simulink model "Iris_DeePC_Control_Gazebo_hyper"  (R2022a)
settings: Solver=VariableStepAuto  StartTime=0.0  StopTime=sim_time  RelTol=1e-3
values from neighbouring files (symbols this model uses):
  accel_g = param.g    [DeePC_main.m]
  DeePC_param = evalin('base', 'DeePC_param')    [DeePC_Optimizer_osqp.m]
  flag_input_transform_nonlinearity = true    [DeePC_main.m]
  K_pitch = param.K_lqr_outer_loop(3,8)    [DeePC_main.m]
  K_roll = param.K_lqr_outer_loop(2,7)    [DeePC_main.m]
  K_yaw = param.K_lqr_outer_loop(4,9)    [DeePC_main.m]
  Ki_xy = 0    [DeePC_main.m]
  Ki_z = 0    [DeePC_main.m]
  Kp_xy = - param.K_lqr_outer_loop(3,1)/param.K_lqr_outer_loop(2,7)    [DeePC_main.m]
  Kp_z = - param.K_lqr_outer_loop(1,3)    [DeePC_main.m]
  Kv_xy = - param.K_lqr_outer_loop(3,4)/param.K_lqr_outer_loop(2,7)    [DeePC_main.m]
  Kv_z = - param.K_lqr_outer_loop(1,6)    [DeePC_main.m]
  mass = param.nrotor_vehicle_mass_for_controller    [DeePC_main.m]
  param = evalin('base', 'param')    [DeePC_Optimizer_osqp.m]    (also in DeePC_main.m = load_crazyflie_parameters(i_aux))
  start_time = 5    [DeePC_main.m]
undefined symbols (not defined in the file or in its folder): DiscIntNeverNeededParam
libraries: simulink x3, Crazyflie_Library x1
settings Model: Creator=ezzat  LastModifiedBy=simao
settings SolverCC: AlgebraicLoopSolver=LineSearch
settings DataIOCC: ReturnWorkspaceOutputs=off
settings DebuggingCC: UnconnectedInputMsg=warning  UnconnectedOutputMsg=warning  UnconnectedLineMsg=warning  SFMachineParentedDataDiag=warning  ArithmeticOperatorsInVariantConditions=warning
settings SFSimCC: CustomCodeUndefinedFunction=UseInterfaceOnly

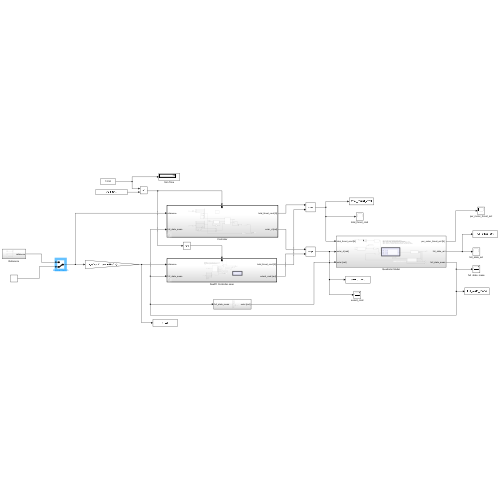
[thumbnail: Simulink's stored preview of the top-level diagram]
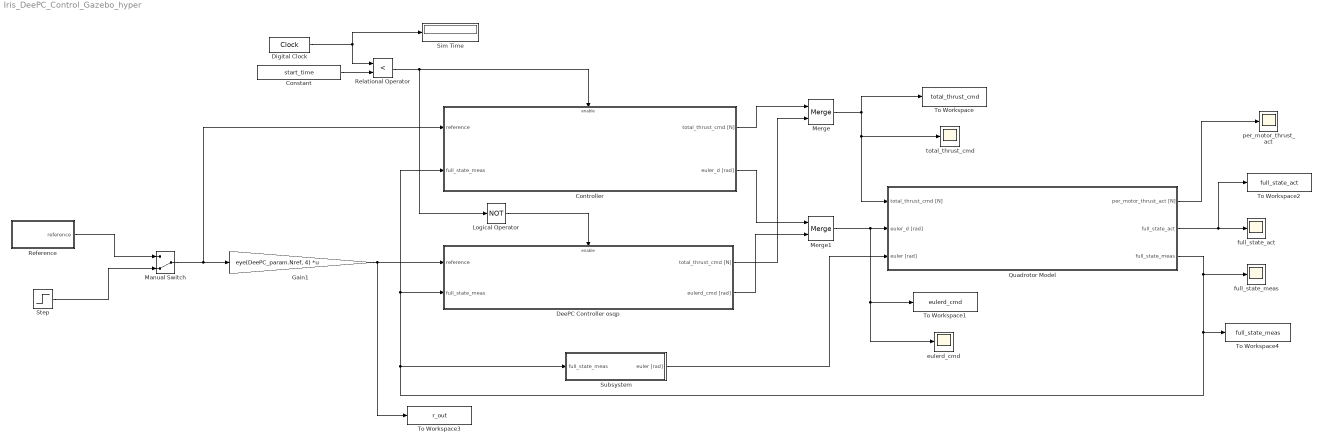
== system Iris_DeePC_Control_Gazebo_hyper ==
  Constant : Constant  Value=start_time
  Controller : Subsystem  AncestorBlock=Crazyflie_Library/LQR_Controller
  DeePC Controller osqp : Subsystem  AncestorBlock=Crazyflie_Library/DeePC_Controller_osqp
  Digital Clock : DigitalClock  SampleTime=param.sample_time_controller_outer
  Gain1 : Gain  Gain=eye(DeePC_param.Nref, 4)  Multiplication=Matrix(K*u)
  Logical Operator : Logic  Operator=NOT  AllPortsSameDT=off  OutDataTypeStr=boolean
  Manual Switch : ManualSwitch  CurrentSetting=0
  Merge : Merge
  Merge1 : Merge
  Quadrotor Model : Subsystem
  Reference : Subsystem
  Relational Operator : RelationalOperator  Operator=<  OutDataTypeStr=boolean  RndMeth=Simplest  InputSameDT=off
  Sim Time : Display
  Step : Step  Time=start_time  Before=[param.nrotor_initial_condition(1:3); param.nrotor_initial_condition(9)]  After=[param.nrotor_final_condition(1:3); param.nrotor_final_condition(9)]  SampleTime=0
  Subsystem : Subsystem
  To Workspace : ToWorkspace  VariableName=total_thrust_cmd  SampleTime=param.sample_time_controller_outer
  To Workspace1 : ToWorkspace  VariableName=eulerd_cmd  SampleTime=param.sample_time_controller_outer
  To Workspace2 : ToWorkspace  VariableName=full_state_act  SampleTime=param.sample_time_controller_outer
  To Workspace3 : ToWorkspace  VariableName=r_out  SampleTime=param.sample_time_controller_outer
  To Workspace4 : ToWorkspace  VariableName=full_state_meas  SampleTime=param.sample_time_controller_outer
  eulerd_cmd : Scope
  full_state_act : Scope
  full_state_meas : Scope
  per_motor_thrust_act : Scope
  total_thrust_cmd : Scope
  wires:
  Quadrotor Model/2(full_state_act) -> To Workspace2/1, full_state_act/1
  Quadrotor Model/3(full_state_meas) -> To Workspace4/1, Controller/2(full_state_meas), DeePC Controller osqp/2(full_state_meas), Subsystem/1(full_state_meas), full_state_meas/1
  Digital Clock/1 -> Sim Time/1, Relational Operator/1
  Constant/1 -> Relational Operator/2
  DeePC Controller osqp/1(total_thrust_cmd [N]) -> Merge/2
  Merge/1 -> Quadrotor Model/1(total_thrust_cmd [N]), total_thrust_cmd/1, To Workspace/1
  Merge1/1 -> Quadrotor Model/2(euler_d [rad]), To Workspace1/1, eulerd_cmd/1
  DeePC Controller osqp/2(eulerd_cmd [rad]) -> Merge1/2
  Logical Operator/1 -> DeePC Controller osqp/Enable
  Quadrotor Model/1("per_motor_thrust_act [N] ") -> per_motor_thrust_act/1
  Gain1/1 -> DeePC Controller osqp/1(reference), To Workspace3/1
  Controller/1(total_thrust_cmd [N]) -> Merge/1
  Controller/2(euler_d [rad]) -> Merge1/1
  Subsystem/1(euler [rad]) -> Quadrotor Model/3(euler [rad])
  Relational Operator/1 -> Controller/Enable, Logical Operator/1
  Manual Switch/1 -> Controller/1(reference), Gain1/1
  Step/1 -> Manual Switch/2
  Reference/1(reference) -> Manual Switch/1

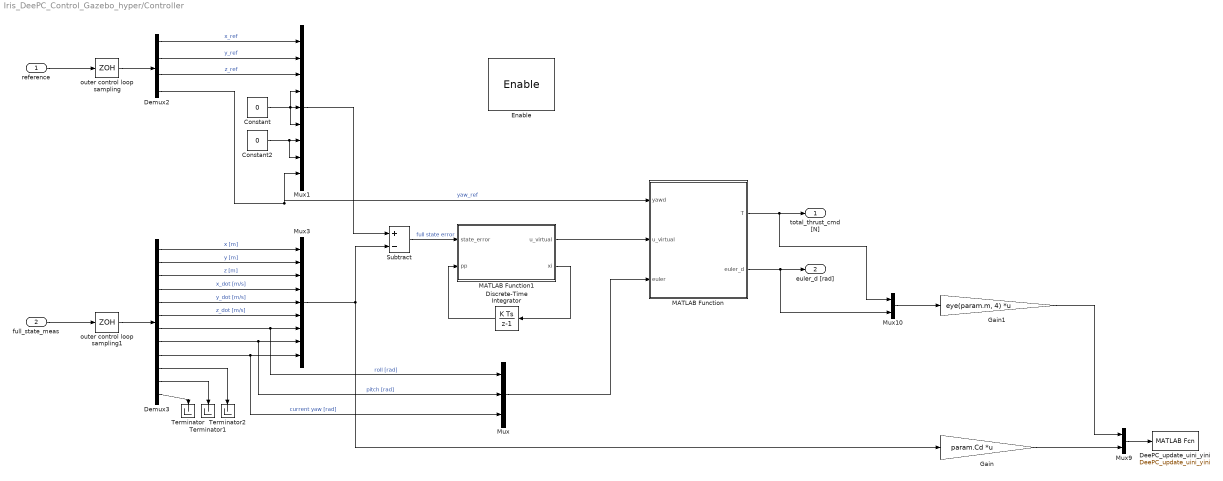
== system Iris_DeePC_Control_Gazebo_hyper/Controller ==
  reference : Inport
  full_state_meas : Inport  Port=2
  Enable : EnablePort
  Constant : Constant  Value=0
  Constant2 : Constant  Value=0
  DeePC_update_uini_yini : MATLABFcn  MATLABFcn=DeePC_update_uini_yini  OutputDimensions=0
  Demux2 : Demux
  Demux3 : Demux  Outputs=12
  Discrete-Time Integrator : DiscreteIntegrator  InitialCondition=[0;0;0]  SampleTime=-1  ICPrevOutput=DiscIntNeverNeededParam  ICPrevScaledInput=DiscIntNeverNeededParam
  Gain : Gain  Gain=param.Cd  Multiplication=Matrix(K*u)
  Gain1 : Gain  Gain=eye(param.m, 4)  Multiplication=Matrix(K*u)
  MATLAB Function : MATLAB Function  TreatAsAtomicUnit=on
  MATLAB Function1 : MATLAB Function  TreatAsAtomicUnit=on
  Mux : Mux  Inputs=3
  Mux1 : Mux  Inputs=9
  Mux10 : Mux  Inputs=2
  Mux3 : Mux  Inputs=9
  Mux9 : Mux  Inputs=2
  Subtract : Sum  Inputs=+-
  Terminator : Terminator
  Terminator1 : Terminator
  Terminator2 : Terminator
  outer control loop sampling : ZeroOrderHold  SampleTime=param.sample_time_controller_outer
  outer control loop sampling1 : ZeroOrderHold  SampleTime=param.sample_time_controller_outer
  total_thrust_cmd [N] : Outport
  euler_d [rad] : Outport  Port=2
  wires:
  Mux3/1 -> Gain/1, Subtract/2
  Demux3/11 -> Terminator1/1
  Demux2/1 -> Mux1/1  "x_ref"
  Demux3/1 -> Mux3/1  "x [m]"
  Demux3/3 -> Mux3/3  "z [m]"
  Demux3/6 -> Mux3/6  "z_dot [m/s]"
  Constant/1 -> Mux1/5, Mux1/4, Mux1/6
  Constant2/1 -> Mux1/8, Mux1/7
  Demux3/2 -> Mux3/2  "y [m]"
  Demux2/4 -> Mux1/9, MATLAB Function/1(yawd)  "yaw_ref"
  Demux3/8 -> Mux3/8, Mux/2  "pitch [rad]"
  Demux3/12 -> Terminator/1
  Demux3/9 -> Mux3/9, Mux/3  "current yaw [rad]"
  Demux3/7 -> Mux/1, Mux3/7  "roll [rad]"
  Demux2/2 -> Mux1/2  "y_ref"
  Demux3/10 -> Terminator2/1
  Demux3/4 -> Mux3/4  "x_dot [m/s]"
  Demux2/3 -> Mux1/3  "z_ref"
  Mux1/1 -> Subtract/1
  Demux3/5 -> Mux3/5  "y_dot [m/s]"
  full_state_meas/1 -> outer control loop sampling1/1
  outer control loop sampling/1 -> Demux2/1
  reference/1 -> outer control loop sampling/1
  outer control loop sampling1/1 -> Demux3/1
  Subtract/1 -> MATLAB Function1/1(state_error)  "full state error"
  MATLAB Function1/2(xi) -> Discrete-Time Integrator/1
  Discrete-Time Integrator/1 -> MATLAB Function1/2(pp)
  MATLAB Function1/1(u_virtual) -> MATLAB Function/2(u_virtual)
  MATLAB Function/1(T) -> total_thrust_cmd [N]/1, Mux10/1
  MATLAB Function/2(euler_d) -> Mux10/2, euler_d [rad]/1
  Mux9/1 -> DeePC_update_uini_yini/1
  Mux10/1 -> Gain1/1
  Gain/1 -> Mux9/2
  Gain1/1 -> Mux9/1
  Mux/1 -> MATLAB Function/3(euler)

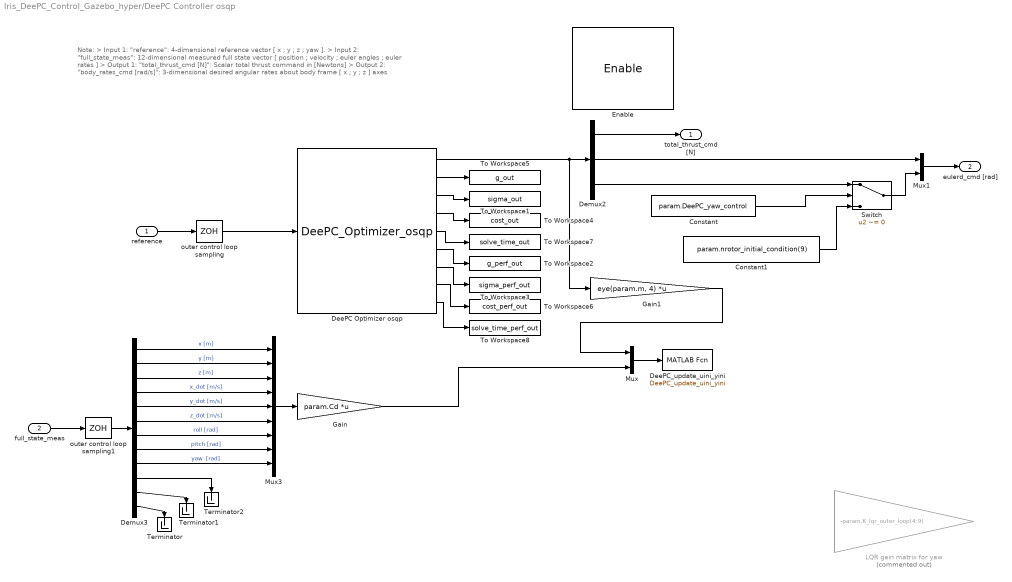
== system Iris_DeePC_Control_Gazebo_hyper/DeePC Controller osqp ==
  note: Note:
      | > Input 1: "reference": 4-dimensional reference vector [ x ; y ; z ; yaw ].
      | > Input 2: "full_state_meas": 12-dimensional measured full state vector [ position ; velocity ; euler angles ; euler rates ]
      | > Output 1: "total_thrust_cmd [N]": Scalar total thrust command in [Newtons]
      | > Output 2: "body_rates_cmd [rad/s]": 3-dimensional desired angular rates about body frame [ x ; y ; z ] axes
  reference : Inport
  full_state_meas : Inport  Port=2
  Enable : EnablePort
  Constant : Constant  Value=param.DeePC_yaw_control
  Constant1 : Constant  Value=param.nrotor_initial_condition(9)
  DeePC Optimizer osqp : Crazyflie_Library/DeePC_Optimizer_osqp  SystemSampleTime=-1  VariantActivationTime=update diagram  Latency=0  AutoFrameSizeCalculation=off
  DeePC_update_uini_yini : MATLABFcn  MATLABFcn=DeePC_update_uini_yini  OutputDimensions=0
  Demux2 : Demux  Outputs=[1 2 1]
  Demux3 : Demux  Outputs=12
  Gain : Gain  Gain=param.Cd  Multiplication=Matrix(K*u)
  Gain1 : Gain  Gain=eye(param.m, 4)  Multiplication=Matrix(K*u)
  LQR gain matrix for yaw : Gain  Commented=on  Gain=-param.K_lqr_outer_loop(4:9)
  Mux : Mux  Inputs=2
  Mux1 : Mux  Inputs=[2 1]
  Mux3 : Mux  Inputs=9
  Switch : Switch  Criteria=u2 ~= 0  SaturateOnIntegerOverflow=off  InputSameDT=off
  Terminator : Terminator
  Terminator1 : Terminator
  Terminator2 : Terminator
  To Workspace1 : ToWorkspace  VariableName=sigma_out  SampleTime=-1
  To Workspace2 : ToWorkspace  VariableName=g_perf_out  SampleTime=-1
  To Workspace3 : ToWorkspace  VariableName=sigma_perf_out  SampleTime=-1
  To Workspace4 : ToWorkspace  VariableName=cost_out  SampleTime=-1
  To Workspace5 : ToWorkspace  VariableName=g_out  SampleTime=-1
  To Workspace6 : ToWorkspace  VariableName=cost_perf_out  SampleTime=-1
  To Workspace7 : ToWorkspace  VariableName=solve_time_out  SampleTime=-1
  To Workspace8 : ToWorkspace  VariableName=solve_time_perf_out  SampleTime=-1
  outer control loop sampling : ZeroOrderHold  SampleTime=param.sample_time_controller_outer
  outer control loop sampling1 : ZeroOrderHold  SampleTime=param.sample_time_controller_outer
  total_thrust_cmd [N] : Outport  VectorParamsAs1DForOutWhenUnconnected=off
  eulerd_cmd [rad] : Outport  Port=2  VectorParamsAs1DForOutWhenUnconnected=off
  wires:
  DeePC Optimizer osqp/7 -> To Workspace3/1
  DeePC Optimizer osqp/4 -> To Workspace4/1
  DeePC Optimizer osqp/3 -> To Workspace1/1
  DeePC Optimizer osqp/8 -> To Workspace6/1
  DeePC Optimizer osqp/6 -> To Workspace2/1
  DeePC Optimizer osqp/5 -> To Workspace7/1
  DeePC Optimizer osqp/9 -> To Workspace8/1
  DeePC Optimizer osqp/2 -> To Workspace5/1
  Gain1/1 -> Mux/1
  Constant/1 -> Switch/2
  Switch/1 -> Mux1/2
  Demux2/3 -> Switch/1
  Demux3/9 -> Mux3/9  "yaw  [rad]"
  Mux1/1 -> eulerd_cmd [rad]/1
  Demux2/2 -> Mux1/1
  DeePC Optimizer osqp/1 -> Demux2/1, Gain1/1
  Gain/1 -> Mux/2
  Mux/1 -> DeePC_update_uini_yini/1
  outer control loop sampling/1 -> DeePC Optimizer osqp/1
  Demux2/1 -> total_thrust_cmd [N]/1
  Mux3/1 -> Gain/1
  outer control loop sampling1/1 -> Demux3/1
  reference/1 -> outer control loop sampling/1
  full_state_meas/1 -> outer control loop sampling1/1
  Demux3/5 -> Mux3/5  "y_dot [m/s]"
  Demux3/4 -> Mux3/4  "x_dot [m/s]"
  Demux3/10 -> Terminator2/1
  Demux3/7 -> Mux3/7  "roll [rad]"
  Demux3/12 -> Terminator/1
  Demux3/8 -> Mux3/8  "pitch [rad]"
  Demux3/2 -> Mux3/2  "y [m]"
  Demux3/6 -> Mux3/6  "z_dot [m/s]"
  Demux3/3 -> Mux3/3  "z [m]"
  Demux3/1 -> Mux3/1  "x [m]"
  Demux3/11 -> Terminator1/1
  Constant1/1 -> Switch/3

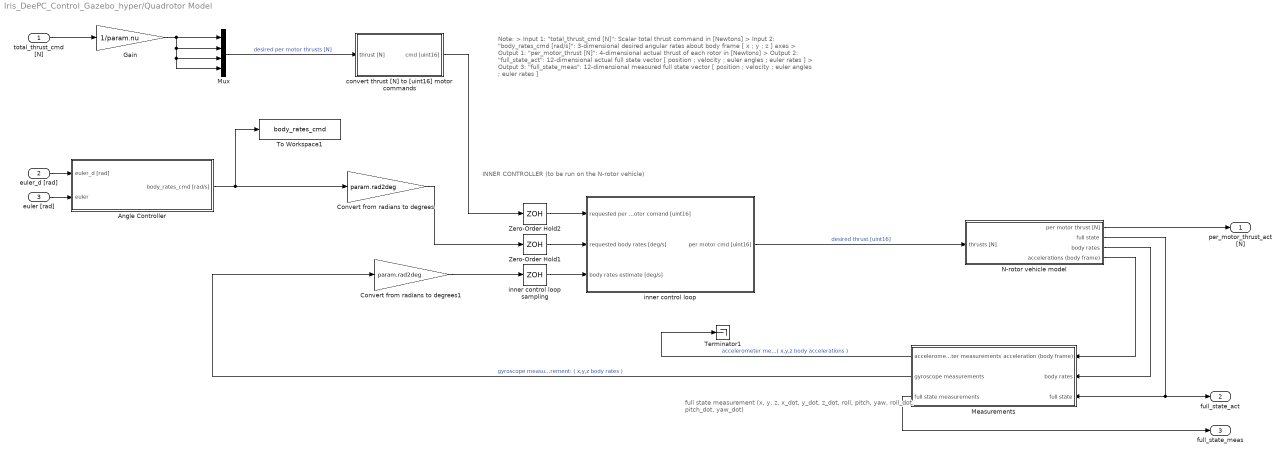
== system Iris_DeePC_Control_Gazebo_hyper/Quadrotor Model ==
  note: INNER CONTROLLER (to be run on the N-rotor vehicle)
  note: full state measurement
      | (x, y, z, x_dot, y_dot, z_dot, roll, pitch, yaw, roll_dot, pitch_dot, yaw_dot)
  note: Note:
      | > Input 1: "total_thrust_cmd [N]": Scalar total thrust command in [Newtons]
      | > Input 2: "body_rates_cmd [rad/s]": 3-dimensional desired angular rates about body frame [ x ; y ; z ] axes
      | > Output 1: "per_motor_thrust [N]": 4-dimensional actual thrust of each rotor in [Newtons]
      | > Output 2: "full_state_act": 12-dimensional actual full state vector [ position ; velocity ; euler angles ; euler rates ]
      | > Output 3: "full_state_meas": 12-dimensional measured full state vector [ position ; velocity ; euler angles ; euler rates ]
  total_thrust_cmd [N] : Inport
  euler_d [rad] : Inport  Port=2
  euler [rad] : Inport  Port=3
  Angle Controller : Subsystem
  Convert from radians to degrees : Gain  Gain=param.rad2deg
  Convert from radians to degrees1 : Gain  Gain=param.rad2deg
  Gain : Gain  Gain=1/param.nu
  Measurements : Subsystem
  Mux : Mux  Inputs=param.nu
  N-rotor vehicle model : Subsystem
  Terminator1 : Terminator
  To Workspace1 : ToWorkspace  VariableName=body_rates_cmd  SampleTime=param.sample_time_controller_outer
  Zero-Order Hold1 : ZeroOrderHold  SampleTime=param.sample_time_controller_inner
  Zero-Order Hold2 : ZeroOrderHold  SampleTime=param.sample_time_controller_inner
  convert thrust [N] to [uint16] motor commands : Subsystem
  inner control loop sampling : ZeroOrderHold  SampleTime=param.sample_time_controller_inner
  inner control loop : Subsystem
  "per_motor_thrust_act [N] " : Outport  VectorParamsAs1DForOutWhenUnconnected=off
  full_state_act : Outport  Port=2  VectorParamsAs1DForOutWhenUnconnected=off
  full_state_meas : Outport  Port=3  VectorParamsAs1DForOutWhenUnconnected=off
  wires:
  Angle Controller/1(body_rates_cmd [rad/s]) -> Convert from radians to degrees/1, To Workspace1/1
  Measurements/2(gyroscope measurements) -> Convert from radians to degrees1/1  "gyroscope measurement: ( x,y,z body rates )"
  inner control loop sampling/1 -> inner control loop/3(body rates estimate [deg/s])
  total_thrust_cmd [N]/1 -> Gain/1
  N-rotor vehicle model/4(accelerations (body frame)) -> Measurements/1(acceleration (body frame))
  Zero-Order Hold2/1 -> inner control loop/1(requested per motor comand [uint16])
  inner control loop/1(per motor cmd [uint16]) -> N-rotor vehicle model/1(thrusts [N])  "desired thrust [uint16]"
  Convert from radians to degrees1/1 -> inner control loop sampling/1
  Measurements/3(full state measurements) -> full_state_meas/1
  N-rotor vehicle model/3(body rates) -> Measurements/2(body rates)
  N-rotor vehicle model/1(per motor thrust [N]) -> "per_motor_thrust_act [N] "/1
  N-rotor vehicle model/2(full state) -> full_state_act/1, Measurements/3(full state)
  Measurements/1(accelerometer measurements) -> Terminator1/1  "accelerometer measurement: ( x,y,z body accelerations )"
  Mux/1 -> convert thrust [N] to [uint16] motor commands/1(thrust [N])  "desired per motor thrusts [N]"
  Convert from radians to degrees/1 -> Zero-Order Hold1/1
  Zero-Order Hold1/1 -> inner control loop/2(requested body rates [deg/s])
  Gain/1 -> Mux/1, Mux/2, Mux/3, Mux/4
  euler [rad]/1 -> Angle Controller/2(euler)
  euler_d [rad]/1 -> Angle Controller/1(euler_d [rad])
  convert thrust [N] to [uint16] motor commands/1(cmd [uint16]) -> Zero-Order Hold2/1

== system Iris_DeePC_Control_Gazebo_hyper/Reference ==
  Step : Step  Time=start_time  Before=[param.nrotor_initial_condition(1:3); param.nrotor_initial_condition(9)]  After=[param.nrotor_final_condition(1:3); param.nrotor_final_condition(9)]  SampleTime=0
  Step1 : Step  Time=start_time+20  Before=[0;0;0;0]  After=[-1;-1;1;0]  SampleTime=0
  Step3 : Step  Time=start_time+40  Before=[0;0;0;0]  After=[1;1;-1;0]  SampleTime=0
  Sum : Sum  Inputs=+++
  reference : Outport
  wires:
  Sum/1 -> reference/1
  Step/1 -> Sum/1
  Step1/1 -> Sum/2
  Step3/1 -> Sum/3

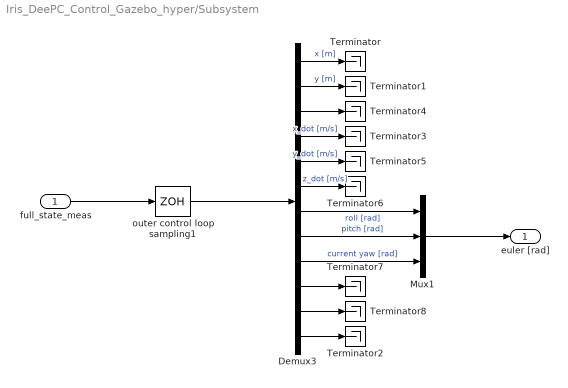
== system Iris_DeePC_Control_Gazebo_hyper/Subsystem ==
  full_state_meas : Inport
  Demux3 : Demux  Outputs=12
  Mux1 : Mux  Inputs=3
  Terminator{,1..8} (9 alike) : Terminator
  outer control loop sampling1 : ZeroOrderHold  SampleTime=param.sample_time_controller_outer
  euler [rad] : Outport
  wires:
  Demux3/7 -> Mux1/1  "roll [rad]"
  outer control loop sampling1/1 -> Demux3/1
  Demux3/8 -> Mux1/2  "pitch [rad]"
  full_state_meas/1 -> outer control loop sampling1/1
  Demux3/9 -> Mux1/3  "current yaw [rad]"
  Mux1/1 -> euler [rad]/1
  Demux3/1 -> Terminator/1  "x [m]"
  Demux3/2 -> Terminator1/1  "y [m]"
  Demux3/3 -> Terminator4/1
  Demux3/4 -> Terminator3/1  "x_dot [m/s]"
  Demux3/5 -> Terminator5/1  "y_dot [m/s]"
  Demux3/6 -> Terminator6/1  "z_dot [m/s]"
  Demux3/10 -> Terminator7/1
  Demux3/11 -> Terminator8/1
  Demux3/12 -> Terminator2/1

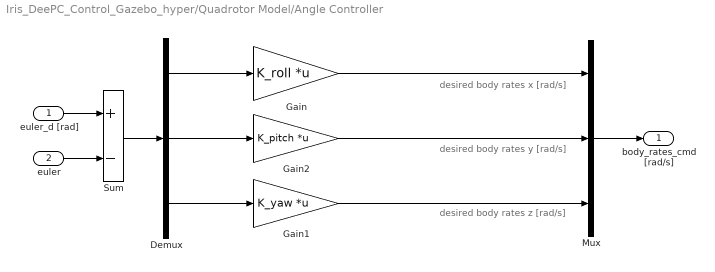
== system Iris_DeePC_Control_Gazebo_hyper/Quadrotor Model/Angle Controller ==
  note: desired body rates x [rad/s]
  note: desired body rates z [rad/s]
  note: desired body rates y [rad/s]
  euler_d [rad] : Inport
  euler : Inport  Port=2
  Demux : Demux  Outputs=3
  Gain : Gain  Gain=K_roll  Multiplication=Matrix(K*u)
  Gain1 : Gain  Gain=K_yaw  Multiplication=Matrix(K*u)
  Gain2 : Gain  Gain=K_pitch  Multiplication=Matrix(K*u)
  Mux : Mux  Inputs=3
  Sum : Sum  Inputs=+-
  body_rates_cmd [rad/s] : Outport
  wires:
  euler_d [rad]/1 -> Sum/1
  euler/1 -> Sum/2
  Demux/2 -> Gain2/1
  Demux/3 -> Gain1/1
  Mux/1 -> body_rates_cmd [rad/s]/1
  Sum/1 -> Demux/1
  Gain2/1 -> Mux/2
  Gain1/1 -> Mux/3
  Gain/1 -> Mux/1
  Demux/1 -> Gain/1

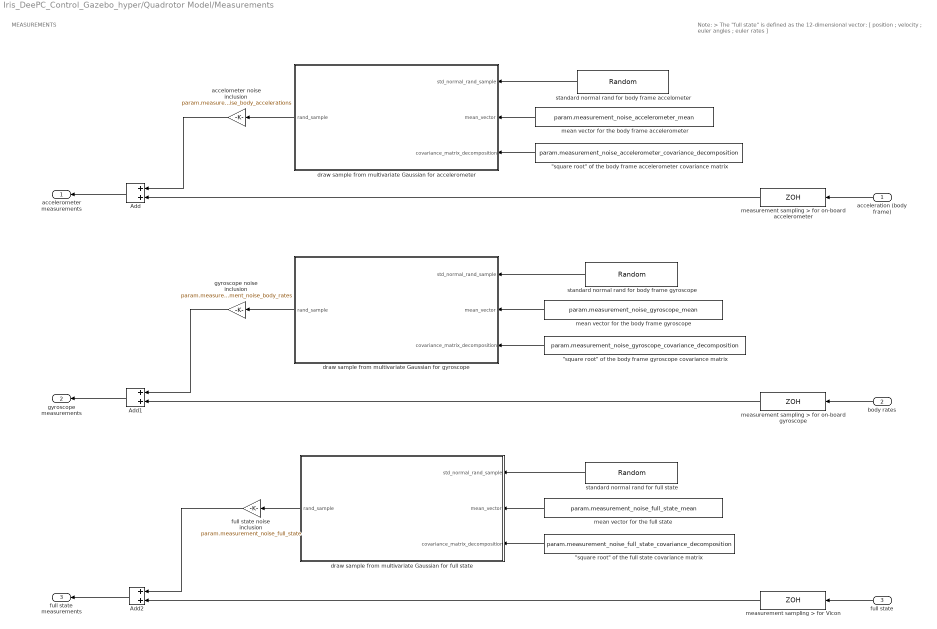
== system Iris_DeePC_Control_Gazebo_hyper/Quadrotor Model/Measurements ==
  note: MEASUREMENTS
  note: Note:
      | > The "full state" is defined as the 12-dimensional vector:
      | [ position ; velocity ; euler angles ; euler rates ]
  acceleration (body frame) : Inport
  body rates : Inport  Port=2
  full state : Inport  Port=3
  "\"square root\" of the body frame accelerometer covariance matrix" : Constant  Value=param.measurement_noise_accelerometer_covariance_decomposition
  "\"square root\" of the body frame gyroscope covariance matrix" : Constant  Value=param.measurement_noise_gyroscope_covariance_decomposition
  "\"square root\" of the full state covariance matrix" : Constant  Value=param.measurement_noise_full_state_covariance_decomposition
  Add : Sum
  Add1 : Sum
  Add2 : Sum
  accelometer noise inclusion : Gain  Gain=param.measurement_noise_body_accelerations
  draw sample from multivariate Gaussian for accelerometer : MATLAB Function  TreatAsAtomicUnit=on
  draw sample from multivariate Gaussian for full state : MATLAB Function  TreatAsAtomicUnit=on
  draw sample from multivariate Gaussian for gyroscope : MATLAB Function  TreatAsAtomicUnit=on
  full state noise inclusion : Gain  Gain=param.measurement_noise_full_state
  gyroscope noise inclusion : Gain  Gain=param.measurement_noise_body_rates
  mean vector for the body frame accelerometer : Constant  Value=param.measurement_noise_accelerometer_mean
  mean vector for the body frame gyroscope : Constant  Value=param.measurement_noise_gyroscope_mean
  mean vector for the full state : Constant  Value=param.measurement_noise_full_state_mean
  measurement sampling > for Vicon : ZeroOrderHold  SampleTime=param.sample_time_measurements_full_state
  measurement sampling > for on-board accelerometer : ZeroOrderHold  SampleTime=param.sample_time_measurements_body_accelerations
  measurement sampling > for on-board gyroscope : ZeroOrderHold  SampleTime=param.sample_time_measurements_body_rates
  standard normal rand for body frame accelometer : RandomNumber  Mean=zeros(size(param.measurement_noise_accelerometer_mean))  Variance=ones(size(param.measurement_noise_accelerometer_mean))  Seed=param.measurement_noise_accelerometer_seed  SampleTime=param.sample_time_measurements_body_accelerations  VectorParams1D=off
  standard normal rand for body frame gyroscope : RandomNumber  Mean=zeros(size(param.measurement_noise_gyroscope_mean))  Variance=ones(size(param.measurement_noise_gyroscope_mean))  Seed=param.measurement_noise_gyroscope_seed  SampleTime=param.sample_time_measurements_body_rates  VectorParams1D=off
  standard normal rand for full state : RandomNumber  Mean=zeros(size(param.measurement_noise_full_state_mean))  Variance=ones(size(param.measurement_noise_full_state_mean))  Seed=param.measurement_noise_full_state_seed  SampleTime=param.sample_time_measurements_full_state  VectorParams1D=off
  accelerometer measurements : Outport  VectorParamsAs1DForOutWhenUnconnected=off
  gyroscope measurements : Outport  Port=2  VectorParamsAs1DForOutWhenUnconnected=off
  full state measurements : Outport  Port=3  VectorParamsAs1DForOutWhenUnconnected=off
  wires:
  Add1/1 -> gyroscope measurements/1
  Add/1 -> accelerometer measurements/1
  "\"square root\" of the body frame accelerometer covariance matrix"/1 -> draw sample from multivariate Gaussian for accelerometer/3(covariance_matrix_decomposition)
  Add2/1 -> full state measurements/1
  standard normal rand for body frame accelometer/1 -> draw sample from multivariate Gaussian for accelerometer/1(std_normal_rand_sample)
  standard normal rand for body frame gyroscope/1 -> draw sample from multivariate Gaussian for gyroscope/1(std_normal_rand_sample)
  measurement sampling > for on-board gyroscope/1 -> Add1/2
  full state noise inclusion/1 -> Add2/1
  draw sample from multivariate Gaussian for full state/1(rand_sample) -> full state noise inclusion/1
  accelometer noise inclusion/1 -> Add/1
  "\"square root\" of the body frame gyroscope covariance matrix"/1 -> draw sample from multivariate Gaussian for gyroscope/3(covariance_matrix_decomposition)
  standard normal rand for full state/1 -> draw sample from multivariate Gaussian for full state/1(std_normal_rand_sample)
  draw sample from multivariate Gaussian for gyroscope/1(rand_sample) -> gyroscope noise inclusion/1
  draw sample from multivariate Gaussian for accelerometer/1(rand_sample) -> accelometer noise inclusion/1
  mean vector for the body frame accelerometer/1 -> draw sample from multivariate Gaussian for accelerometer/2(mean_vector)
  measurement sampling > for on-board accelerometer/1 -> Add/2
  gyroscope noise inclusion/1 -> Add1/1
  mean vector for the body frame gyroscope/1 -> draw sample from multivariate Gaussian for gyroscope/2(mean_vector)
  mean vector for the full state/1 -> draw sample from multivariate Gaussian for full state/2(mean_vector)
  "\"square root\" of the full state covariance matrix"/1 -> draw sample from multivariate Gaussian for full state/3(covariance_matrix_decomposition)
  measurement sampling > for Vicon/1 -> Add2/2
  body rates/1 -> measurement sampling > for on-board gyroscope/1
  acceleration (body frame)/1 -> measurement sampling > for on-board accelerometer/1
  full state/1 -> measurement sampling > for Vicon/1

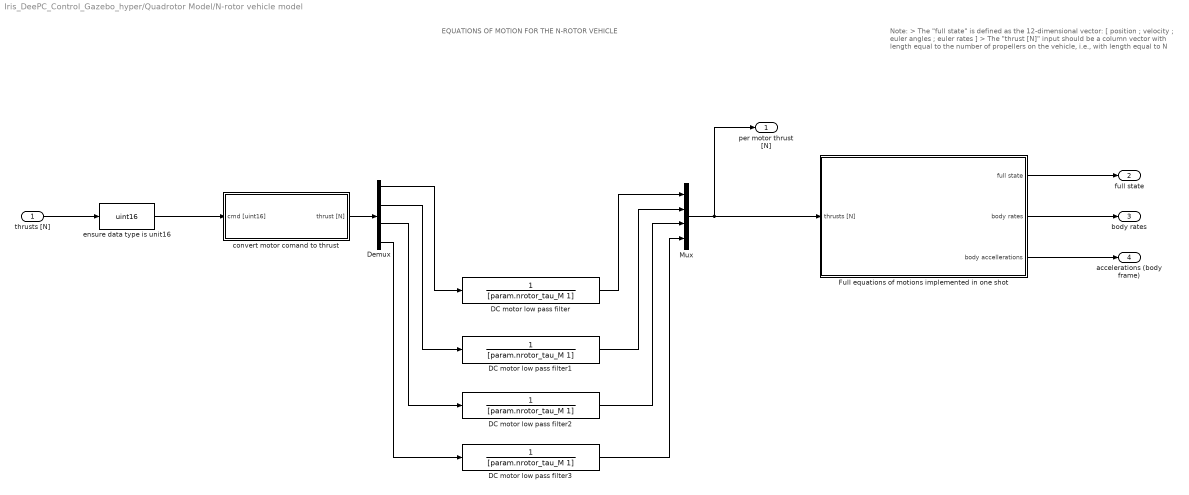
== system Iris_DeePC_Control_Gazebo_hyper/Quadrotor Model/N-rotor vehicle model ==
  note: EQUATIONS OF MOTION FOR THE N-ROTOR VEHICLE
  note: Note:
      | > The "full state" is defined as the 12-dimensional vector:
      | [ position ; velocity ; euler angles ; euler rates ]
      | > The "thrust [N]" input should be a column vector with
      | length equal to the number of propellers on the vehicle,
      | i.e., with length equal to N
  thrusts [N] : Inport
  DC motor low pass filter{,1..3} (4 alike) : TransferFcn  Denominator=[param.nrotor_tau_M 1]
  Demux : Demux
  Full equations of motions implemented in one shot : Subsystem
  Mux : Mux
  convert motor comand to thrust : Subsystem
  ensure data type is unit16 : DataTypeConversion  OutDataTypeStr=uint16  SaturateOnIntegerOverflow=off  RndMeth=Floor
  per motor thrust [N] : Outport  VectorParamsAs1DForOutWhenUnconnected=off
  full state : Outport  Port=2  VectorParamsAs1DForOutWhenUnconnected=off
  body rates : Outport  Port=3  VectorParamsAs1DForOutWhenUnconnected=off
  accelerations (body frame) : Outport  Port=4  VectorParamsAs1DForOutWhenUnconnected=off
  wires:
  DC motor low pass filter/1 -> Mux/1
  Demux/1 -> DC motor low pass filter/1
  DC motor low pass filter1/1 -> Mux/2
  Demux/2 -> DC motor low pass filter1/1
  DC motor low pass filter2/1 -> Mux/3
  Demux/3 -> DC motor low pass filter2/1
  DC motor low pass filter3/1 -> Mux/4
  Demux/4 -> DC motor low pass filter3/1
  Mux/1 -> Full equations of motions implemented in one shot/1(thrusts [N]), per motor thrust [N]/1
  convert motor comand to thrust/1(thrust [N]) -> Demux/1
  ensure data type is unit16/1 -> convert motor comand to thrust/1(cmd [uint16])
  Full equations of motions implemented in one shot/3(body accellerations) -> accelerations (body frame)/1
  Full equations of motions implemented in one shot/2(body rates) -> body rates/1
  Full equations of motions implemented in one shot/1(full state) -> full state/1
  thrusts [N]/1 -> ensure data type is unit16/1

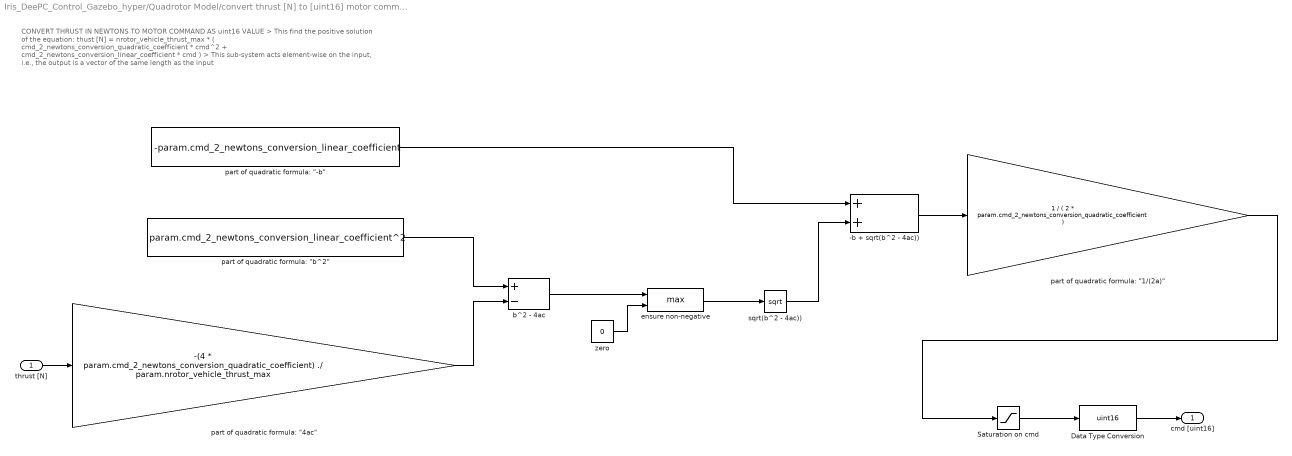
== system Iris_DeePC_Control_Gazebo_hyper/Quadrotor Model/convert thrust [N] to [uint16] motor commands ==
  note: CONVERT THRUST IN NEWTONS TO MOTOR COMMAND AS uint16 VALUE
      | > This find the positive solution of the equation:
      | thust [N] = nrotor_vehicle_thrust_max * ( cmd_2_newtons_conversion_quadratic_coefficient * cmd^2 + cmd_2_newtons_conversion_linear_coefficient * cmd )
      |
      | > This sub-system acts element-wise on the input, i.e., the output is a vector of the same length as the input
  thrust [N] : Inport
  -b + sqrt(b^2 - 4ac)) : Sum
  Data Type Conversion : DataTypeConversion  OutDataTypeStr=uint16  SaturateOnIntegerOverflow=off  RndMeth=Floor
  Saturation on cmd : Saturate  UpperLimit=param.cmd_max  LowerLimit=param.cmd_min  ZeroCross=off
  b^2 - 4ac : Sum  Inputs=+-
  ensure non-negative : MinMax  Function=max  Inputs=2
  "part of quadratic formula: \"-b\"" : Constant  Value=-param.cmd_2_newtons_conversion_linear_coefficient
  "part of quadratic formula: \"1/(2a)\"" : Gain  Gain=1 / ( 2 * param.cmd_2_newtons_conversion_quadratic_coefficient )
  "part of quadratic formula: \"4ac\"" : Gain  Gain=-(4 * param.cmd_2_newtons_conversion_quadratic_coefficient) ./ param.nrotor_vehicle_thrust_max
  "part of quadratic formula: \"b^2\"" : Constant  Value=param.cmd_2_newtons_conversion_linear_coefficient^2
  sqrt(b^2 - 4ac)) : Sqrt
  zero : Constant  Value=0
  cmd [uint16] : Outport  VectorParamsAs1DForOutWhenUnconnected=off
  wires:
  zero/1 -> ensure non-negative/2
  "part of quadratic formula: \"1/(2a)\""/1 -> Saturation on cmd/1
  -b + sqrt(b^2 - 4ac))/1 -> "part of quadratic formula: \"1/(2a)\""/1
  sqrt(b^2 - 4ac))/1 -> -b + sqrt(b^2 - 4ac))/2
  "part of quadratic formula: \"-b\""/1 -> -b + sqrt(b^2 - 4ac))/1
  ensure non-negative/1 -> sqrt(b^2 - 4ac))/1
  b^2 - 4ac/1 -> ensure non-negative/1
  "part of quadratic formula: \"b^2\""/1 -> b^2 - 4ac/1
  "part of quadratic formula: \"4ac\""/1 -> b^2 - 4ac/2
  Data Type Conversion/1 -> cmd [uint16]/1
  Saturation on cmd/1 -> Data Type Conversion/1
  thrust [N]/1 -> "part of quadratic formula: \"4ac\""/1

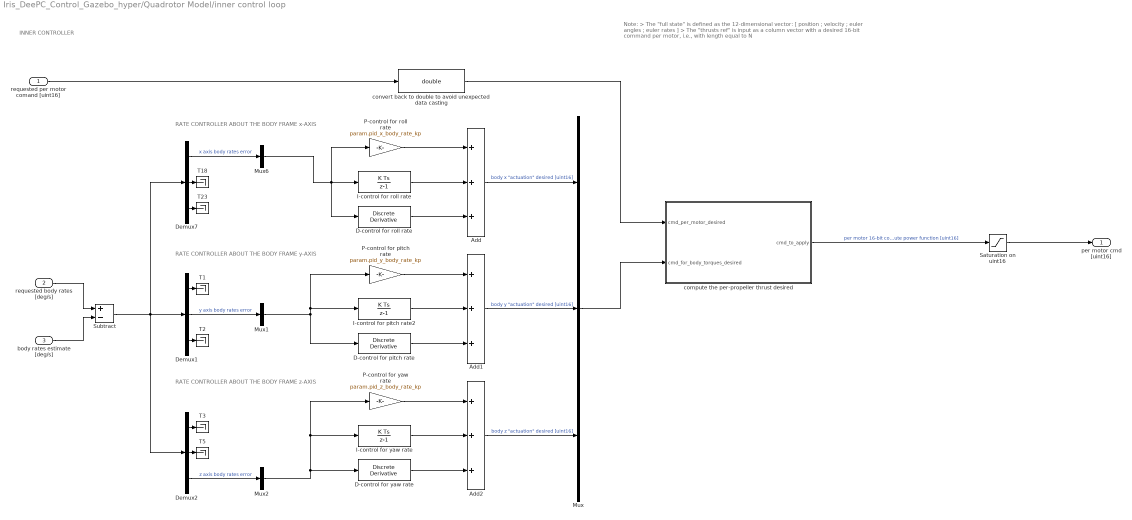
== system Iris_DeePC_Control_Gazebo_hyper/Quadrotor Model/inner control loop ==
  note: Note:
      | > The "full state" is defined as the 12-dimensional vector:
      | [ position ; velocity ; euler angles ; euler rates ]
      | > The "thrusts ref" is input as a column vector with a desired
      | 16-bit command per motor, i.e., with length equal to N
  note: INNER CONTROLLER
  note: RATE CONTROLLER ABOUT THE BODY FRAME x-AXIS
  note: RATE CONTROLLER ABOUT THE BODY FRAME y-AXIS
  note: RATE CONTROLLER ABOUT THE BODY FRAME z-AXIS
  requested per motor comand [uint16] : Inport
  requested body rates [deg/s] : Inport  Port=2
  body rates estimate [deg/s] : Inport  Port=3
  Add : Sum  Inputs=+++
  Add1 : Sum  Inputs=+++
  Add2 : Sum  Inputs=+++
  D-control for pitch rate : simulink/Discrete/Discrete Derivative  gainval=param.pid_y_body_rate_kd  ICPrevScaledInput=0.0  OutMin=[]  OutMax=[]  OutDataType=fixdt(1, 16)  OutScaling=2^-10  DoSatur=off
  D-control for roll rate : simulink/Discrete/Discrete Derivative  gainval=param.pid_x_body_rate_kd  ICPrevScaledInput=0.0  OutMin=[]  OutMax=[]  OutDataType=fixdt(1, 16)  OutScaling=2^-10  DoSatur=off
  D-control for yaw rate : simulink/Discrete/Discrete Derivative  gainval=param.pid_z_body_rate_kd  ICPrevScaledInput=0.0  OutMin=[]  OutMax=[]  OutDataType=fixdt(1, 16)  OutScaling=2^-10  DoSatur=off
  Demux1 : Demux  Outputs=3
  Demux2 : Demux  Outputs=3
  Demux7 : Demux  Outputs=3
  I-control for pitch rate2 : DiscreteIntegrator  gainval=param.pid_y_body_rate_ki  SampleTime=-1  LimitOutput=on  UpperSaturationLimit=param.pid_y_body_rate_integrator_limit  LowerSaturationLimit=-param.pid_y_body_rate_integrator_limit  ICPrevOutput=DiscIntNeverNeededParam  ICPrevScaledInput=DiscIntNeverNeededParam
  I-control for roll rate : DiscreteIntegrator  gainval=param.pid_x_body_rate_ki  SampleTime=-1  LimitOutput=on  UpperSaturationLimit=param.pid_x_body_rate_integrator_limit  LowerSaturationLimit=-param.pid_x_body_rate_integrator_limit  ICPrevOutput=DiscIntNeverNeededParam  ICPrevScaledInput=DiscIntNeverNeededParam
  I-control for yaw rate : DiscreteIntegrator  gainval=param.pid_z_body_rate_ki  SampleTime=-1  LimitOutput=on  UpperSaturationLimit=param.pid_x_body_rate_integrator_limit  LowerSaturationLimit=-param.pid_x_body_rate_integrator_limit  ICPrevOutput=DiscIntNeverNeededParam  ICPrevScaledInput=DiscIntNeverNeededParam
  Mux : Mux  Inputs=3
  Mux1 : Mux  Inputs=1
  Mux2 : Mux  Inputs=1
  Mux6 : Mux  Inputs=1
  P-control for pitch rate : Gain  Gain=param.pid_y_body_rate_kp
  P-control for roll rate : Gain  Gain=param.pid_x_body_rate_kp
  P-control for yaw rate : Gain  Gain=param.pid_z_body_rate_kp
  Saturation on uint16 : Saturate  UpperLimit=param.cmd_max  LowerLimit=param.cmd_min  ZeroCross=off
  Subtract : Sum  Inputs=+-
  T{1..3,5,18,23} (6 alike) : Terminator
  compute the per-propeller thrust desired : MATLAB Function  TreatAsAtomicUnit=on
  convert back to double to avoid unexpected data casting : DataTypeConversion  OutDataTypeStr=double  SaturateOnIntegerOverflow=off  RndMeth=Floor
  per motor cmd [uint16] : Outport  VectorParamsAs1DForOutWhenUnconnected=off
  wires:
  I-control for yaw rate/1 -> Add2/2
  P-control for yaw rate/1 -> Add2/1
  D-control for yaw rate/1 -> Add2/3
  Mux1/1 -> I-control for pitch rate2/1, P-control for pitch rate/1, D-control for pitch rate/1
  D-control for pitch rate/1 -> Add1/3
  I-control for pitch rate2/1 -> Add1/2
  P-control for pitch rate/1 -> Add1/1
  D-control for roll rate/1 -> Add/3
  I-control for roll rate/1 -> Add/2
  P-control for roll rate/1 -> Add/1
  Demux2/2 -> T5/1
  Mux2/1 -> D-control for yaw rate/1, P-control for yaw rate/1, I-control for yaw rate/1
  Demux2/1 -> T3/1
  Demux2/3 -> Mux2/1  "z axis body rates error"
  Demux1/1 -> T1/1
  Demux1/3 -> T2/1
  Demux1/2 -> Mux1/1  "y axis body rates error"
  Demux7/1 -> Mux6/1  "x axis body rates error"
  Demux7/3 -> T23/1
  Mux6/1 -> D-control for roll rate/1, I-control for roll rate/1, P-control for roll rate/1
  Demux7/2 -> T18/1
  Saturation on uint16/1 -> per motor cmd [uint16]/1
  Mux/1 -> compute the per-propeller thrust desired/2(cmd_for_body_torques_desired)
  Subtract/1 -> Demux7/1, Demux1/1, Demux2/1
  Add2/1 -> Mux/3  "body z \"actuation\" desired [uint16]"
  Add1/1 -> Mux/2  "body y \"actuation\" desired [uint16]"
  Add/1 -> Mux/1  "body x \"actuation\" desired [uint16]"
  requested body rates [deg/s]/1 -> Subtract/1
  requested per motor comand [uint16]/1 -> convert back to double to avoid unexpected data casting/1
  body rates estimate [deg/s]/1 -> Subtract/2
  compute the per-propeller thrust desired/1(cmd_to_apply) -> Saturation on uint16/1  "per motor 16-bit command after distribute power function [uint16]"
  convert back to double to avoid unexpected data casting/1 -> compute the per-propeller thrust desired/1(cmd_per_motor_desired)

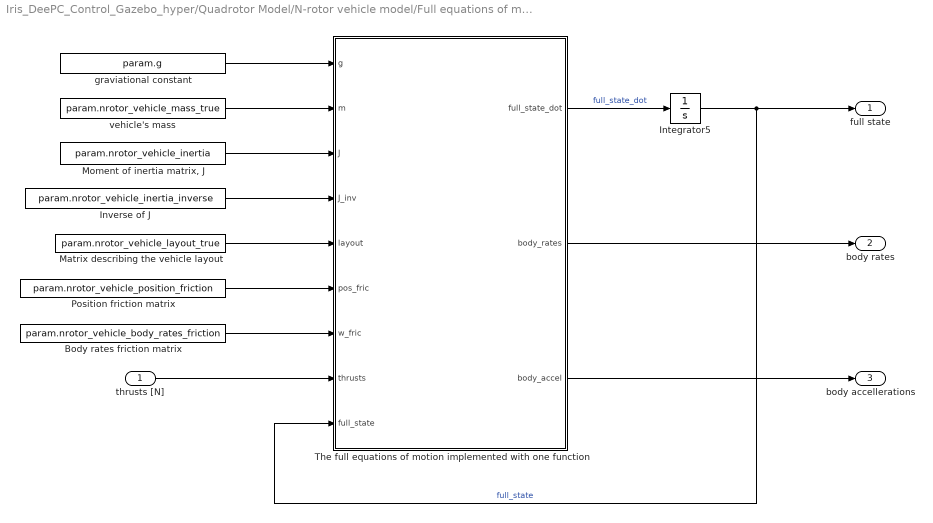
== system Iris_DeePC_Control_Gazebo_hyper/Quadrotor Model/N-rotor vehicle model/Full equations of motions implemented in one shot ==
  thrusts [N] : Inport
  Body rates friction matrix : Constant  Value=param.nrotor_vehicle_body_rates_friction
  Integrator5 : Integrator  InitialCondition=param.nrotor_initial_condition
  Inverse of J : Constant  Value=param.nrotor_vehicle_inertia_inverse
  Matrix describing the vehicle layout : Constant  Value=param.nrotor_vehicle_layout_true
  "Moment of inertia matrix, J" : Constant  Value=param.nrotor_vehicle_inertia
  Position friction matrix : Constant  Value=param.nrotor_vehicle_position_friction
  The full equations of motion implemented with one function : MATLAB Function  TreatAsAtomicUnit=on
  graviational constant : Constant  Value=param.g
  vehicle's mass : Constant  Value=param.nrotor_vehicle_mass_true
  full state : Outport  VectorParamsAs1DForOutWhenUnconnected=off
  body rates : Outport  Port=2  VectorParamsAs1DForOutWhenUnconnected=off
  body accellerations : Outport  Port=3  VectorParamsAs1DForOutWhenUnconnected=off
  wires:
  Body rates friction matrix/1 -> The full equations of motion implemented with one function/7(w_fric)
  Position friction matrix/1 -> The full equations of motion implemented with one function/6(pos_fric)
  "Moment of inertia matrix, J"/1 -> The full equations of motion implemented with one function/3(J)
  vehicle's mass/1 -> The full equations of motion implemented with one function/2(m)
  Inverse of J/1 -> The full equations of motion implemented with one function/4(J_inv)
  Integrator5/1 -> The full equations of motion implemented with one function/9(full_state), full state/1  "full_state"
  The full equations of motion implemented with one function/2(body_rates) -> body rates/1
  thrusts [N]/1 -> The full equations of motion implemented with one function/8(thrusts)
  graviational constant/1 -> The full equations of motion implemented with one function/1(g)
  The full equations of motion implemented with one function/3(body_accel) -> body accellerations/1
  Matrix describing the vehicle layout/1 -> The full equations of motion implemented with one function/5(layout)
  The full equations of motion implemented with one function/1(full_state_dot) -> Integrator5/1  "full_state_dot"

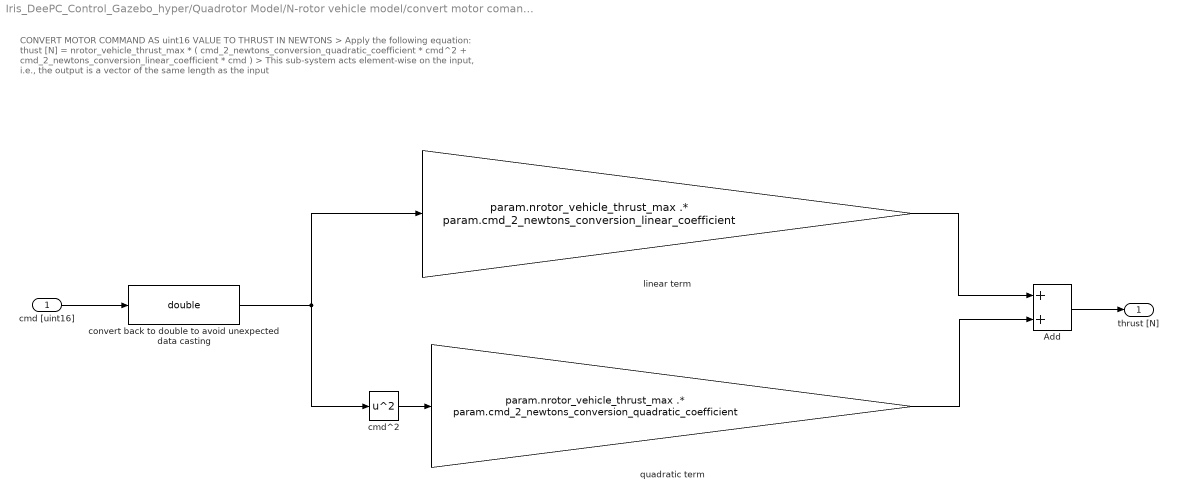
== system Iris_DeePC_Control_Gazebo_hyper/Quadrotor Model/N-rotor vehicle model/convert motor comand to thrust ==
  note: CONVERT MOTOR COMMAND AS uint16 VALUE TO THRUST IN NEWTONS
      | > Apply the following equation:
      | thust [N] = nrotor_vehicle_thrust_max * ( cmd_2_newtons_conversion_quadratic_coefficient * cmd^2 + cmd_2_newtons_conversion_linear_coefficient * cmd )
      |
      | > This sub-system acts element-wise on the input, i.e., the output is a vector of the same length as the input
  cmd [uint16] : Inport
  Add : Sum
  cmd^2 : Math  Operator=square  SignedPower=on
  convert back to double to avoid unexpected data casting : DataTypeConversion  OutDataTypeStr=double  SaturateOnIntegerOverflow=off  RndMeth=Floor
  linear term : Gain  Gain=param.nrotor_vehicle_thrust_max .* param.cmd_2_newtons_conversion_linear_coefficient
  quadratic term : Gain  Gain=param.nrotor_vehicle_thrust_max .* param.cmd_2_newtons_conversion_quadratic_coefficient
  thrust [N] : Outport  VectorParamsAs1DForOutWhenUnconnected=off
  wires:
  convert back to double to avoid unexpected data casting/1 -> cmd^2/1, linear term/1
  Add/1 -> thrust [N]/1
  cmd [uint16]/1 -> convert back to double to avoid unexpected data casting/1
  linear term/1 -> Add/1
  quadratic term/1 -> Add/2
  cmd^2/1 -> quadratic term/1

== matlab function Iris_DeePC_Control_Gazebo_hyper/Quadrotor Model/N-rotor vehicle model/Full equations of motions implemented in one shot/The full equations of motion implemented with one function ==
  data: g input; full_state_dot output; m input; J input; J_inv input; layout input; pos_fric input; w_fric input; thrusts input; full_state input; body_rates output; body_accel output
function [full_state_dot,body_rates,body_accel] = fcn_eom(g,m,J,J_inv,layout,pos_fric,w_fric,thrusts,full_state)
% The "full_state_dot" return argument is a column vector with 12 elements
%full_state_dot = zeros(12,1);

% ----------------------------------------------------------------------- %
% DESCRIPTION:
% This function implements the full equation of motion in one function to
% simplify the exposition.
%
%
% INPUT ARGUMENTS:
% m
% > This is the mass of the vehicle, in units of kilograms
%
% g
% > This is the acceleration due to gravity (typically 9.81), in units of
%   meters per second squared
%
% J
% > This is the moment of inertia matrix of the vehicle (it should be a
%   3-by3 matrix), the units of each element is kilogram meters squared
%
% J_inv
% > This is the inverse of the momement of inertia matrix, it is not
%   compute in this script to reduce the simulation run time slightly
%
% layout
% > This is a matrix that specifies the layout via the following format:
% nrotor_vehicle_layout = [...
%       x_1  ,  x_2  ,  ...  ,  x_{N-1}  ,  x_{N}  ;...
%       y_1  ,  y_2  ,  ...  ,  y_{N-1}  ,  y_{N}  ;...
%       c_1  ,  c_2  ,  ...  ,  c_{N-1}  ,  c_{N}   ...
%   ];
% where:
%   > x_i   is the x coordinate of propeller "i" relative to the CoG
%   > y_i   is the y coordinate of propeller "i" relative to the CoG
%   > c_i   is the thurst to torque coefficient of the propeller, with the
%           sign used to indicate the propeller's direction of rotation,
%           +ve indicates clock-wise propeller rotation.
%
% thrusts
% > This is a colulmn vector with length equal to the number of propellers
%   on the N-rotor vehicle, and each element represents the thrust force in
%   Newtons being produced by the respective propeller
%
% full_state
% > This is a vector of length 12 and is order as:
%   full_state[1:3]     the x,y,z posiiton of the body frame origin
%                       expressed in inertial frame coordinates, in units
%                       of [meters].
%
%   full_state[4:6]     the x,y,z linear velocity of the body frame origin
%                       expressed in inertial frame coordinates, in units
%                       of [meters per second].
%
%   full_state[7:9]     the roll, pitch, and yaw intrinsic Euler angles
%                       respectively, in units of [radians].
%
%   full_state[10:12]   the angular velocity of the roll, pitch, and yaw
%                       intrinsic Euler angles respectively, in units of
%                       [radians per second].
%
% pos_fric
% > This is a 3x3 matrix with friction coefficients for x, y, and z
% velocities. It implements a primitive linear friction model.
%
% w_fric
% > This is a 3x3 matrix with friction coefficients for body rates. It
% implements a primitive linear friction model.
%
%
% RETURN ARGUMENTS:
% full_state_dot
% > This is a vector of length 12 and is ordered as:
%   full_state_dot[1:3]
%      - This is position dot and is taken directly as full_state[4:6]
%
%   full_state_dot[4:6]
%      - This is the position double dot and is computed using the equation
%        of motion for transaltion, it has units of [meters per second
%        squared]
%
%   full_state_dot[7:9]
%      - This is the angular velocity of the intrinsic Euler angles and is
%        taken directly as full_state[10:12]
%
%   full_state_dot[10:12]
%      - This is the angular accelerations of the intrinsic Euler angles
%        and is computed using the equation of motion for Euler angle
%        rotations, it has units of [radians per second squared]
%
% body_rates
% > This is a vector of length 3, each element represents the angular
%   velocity of the body frame as measured about the body frame's
%   coordinate axes, i.e., this is exactly what is measured by a typical
%   strap-down Inertial Measurement Unit (IMU) that is attached to the body
%   of most all flying vehicles. It is computed directly from the "psi_dot"
%   by that is extracted from the "full_state" by applying the
%   transformation matrix "T". It has units of [radians per second];
%
% body_accel
% > This is a vector of length 3, each element represents the linear
%   accelerations of the body frame as measured along the body frame's
%   coordinate axes, i.e., this is exctly what is measured by a typical
%   strap-down Inertial Measurement Unit (IMU). It is computed directly
%   from the "pos_double_dot" by applying the rotation matrix from inertial
%   to body frame. It has units of [meters per second squared].
%
%
% DATA FORMAT ASSUMPTIONS:
% > That the "p" is ordered as:
%   p = [ x ; y ; z ];
% > And equivalently that the "psi_dot" is ordered as:
%   p_dot = [ x_dot ; y_dot ; z_dot ];
% > That the "psi" is ordered as:
%   psi = [ roll ; pitch ; yaw ];
% > And equivalently that the "psi_dot" is ordered as:
%   psi_dot = [ roll_dot ; pitch_dot ; yaw_dot ];
% > That the "w" is ordered as:
%   w = [ w_x ; w_y ; w_z ];
%
% ----------------------------------------------------------------------- %


% Extract the components of the full state
%pos      =  full_state(1:3);
pos_dot  =  full_state(4:6);
psi      =  full_state(7:9);
psi_dot  =  full_state(10:12);


% Extract each Euler angles
r  =  psi(1);  % Roll
p  =  psi(2);  % Pitch
y  =  psi(3);  % Yaw


% Extract each Euler anglular rates
rdot  =  psi_dot(1);  % Roll  angular velocity
pdot  =  psi_dot(2);  % Pitch angular velocity
%ydot  =  psi_dot(3); % Yaw   angular velocity, not needed


% Compute the rotation matrix from body frame to inertial frame:
R_B2I = [...
         cos(y)*cos(p)  ,  cos(y)*sin(p)*sin(r)-sin(y)*cos(r)  ,  cos(y)*sin(p)*cos(r)+sin(y)*sin(r)  ;...
         sin(y)*cos(p)  ,  sin(y)*sin(p)*sin(r)+cos(y)*cos(r)  ,  sin(y)*sin(p)*cos(r)-cos(y)*sin(r)  ;...
        -sin(p)         ,  cos(p)*sin(r)                       ,  cos(p)*cos(r)                        ...
    ];


% Compute the T matrix:
T = [...
        1  ,  0       ,  -sin(p)         ;...
        0  ,  cos(r)  ,   sin(r)*cos(p)  ;...
        0  , -sin(r)  ,   cos(r)*cos(p)   ...
    ];


% Compute the T inverse matrix:
T_inv = [...
        1  ,  sin(r)*tan(p)  ,   cos(r)*tan(p)  ;...
        0  ,  cos(r)         ,  -sin(r)         ;...
        0  ,  sin(r)*sec(p)  ,   cos(r)*sec(p)   ...
    ];


% Compute the time derivative of the T matrix:
T_dot = [...
        0  ,   0            ,  -pdot*cos(p)                            ;...
        0  ,  -rdot*sin(r)  ,   rdot*cos(r)*cos(p)-pdot*sin(r)*sin(p)  ;...
        0  ,  -rdot*cos(r)  ,  -rdot*sin(r)*cos(p)-pdot*cos(r)*sin(p)   ...
    ];


% Implement the equation of motion for translation
pos_double_dot = (-1/m) .* ( R_B2I * [0;0;sum(thrusts(:))] ) + [0;0;g]...
    - transpose(R_B2I)*pos_fric*R_B2I * pos_dot;


% Compute the body rates from the Euler angluar rates
w = T * psi_dot;


% Implement the equation of motion for body frame rotations
% w_dot = J_inv * ( [layout(2,:);-layout(1,:);layout(3,:)] * thrusts - cross( w , J*w ) )...
%     - w_fric * w;

w_dot = J_inv * ( [layout(1,:);layout(2,:);layout(3,:)] * thrusts - cross( w , J*w ) )...
    - w_fric * w;

% Implement the equation of motion for Euler angle rotations
psi_double_dot = T_inv * ( w_dot - T_dot * psi_dot );


% Put together the "full_state_dot" return variable
full_state_dot = [...
        pos_dot ;...
        pos_double_dot ;...
        psi_dot ;...
        psi_double_dot ...
    ];


% Put together the "body_rates" return variable
body_rates = w;


% Finally compute the accelerations in the body frame
% > by "simply" rotating the inertial frame linear accelerations, i.e.,
%   "pos_double_dot", from the inertial frame into the body frame
body_accel = transpose(R_B2I) * pos_double_dot - cross(w, transpose(R_B2I) * pos_dot);


end

== matlab function Iris_DeePC_Control_Gazebo_hyper/Quadrotor Model/inner control loop/compute the per-propeller thrust desired ==
  data: cmd_per_motor_desired input; cmd_for_body_torques_desired input; cmd_to_apply output; inv_M parameter
function cmd_to_apply = distribute_power( cmd_per_motor_desired , cmd_for_body_torques_desired,  inv_M)
% ----------------------------------------------------------------------- %
% DESCRIPTION:
% This function computes the uint16 command to apply to each motor as per
% the code that runs "on-board" on the Crazyflie's firmware
%
%
% INPUT ARGUMENTS:
%
% cmd_per_motor_desired [uint16]
% > This is a colulmn vector with length equal to the number of propellers
%   on the Crazyflie, i.e., 4, and each element represents the "baseline"
%   16-bit command that should be requested from the Crazyflie, as
%   requested by the outer loop controller.
%
% cmd_for_body_torques_desired [uint16]
% > This is the "actuation" uint16 command that comes directly from the
%   output of the Crazyflie's body rate PID controllers running in the
%   firmware. This value of command has already been adjust for the
%   dimensions of the Crazyflie, and the pattern for distributing the
%   command across the motor is provided in the exercise sheet.
%
%
% RETURN ARGUMENTS:
% % cmd_to_apply [uint16]
% > This is a colulmn vector with length equal to the number of propellers
%   on the Crazyflie, i.e., 4, and each element represents the 16-bit
%   command that will be requested from the motors
%
%
% DATA FORMAT ASSUMPTIONS:
% > the "cmd_per_motor_desired" vector is such when applied, the static
%   thrusts exert no torque about the body frame axes
%
% ----------------------------------------------------------------------- %


% Get the uint16 commands into a separate variable for each motor
cmd1 = cmd_per_motor_desired(1);
cmd2 = cmd_per_motor_desired(2);
cmd3 = cmd_per_motor_desired(3);
cmd4 = cmd_per_motor_desired(4);
% 
% 
% % Get the desired body torques uint16 commands into a separate variable for
% % the "uint16 command torque" desired about each of the body frame axes
% r = cmd_for_body_torques_desired(1) / 2;
% p = cmd_for_body_torques_desired(2) / 2;
% y = cmd_for_body_torques_desired(3);
% 
% 
% % These variable names have been used to partially match the code from the
% % Crazyflie firmware:
% % r  -  where "r" stands for roll, this is the "uint16 command torque" to
% %       apply about the body-frame's x-axis, i.e., the roll-axis
% % p  -  where "p" stands for pitch, this is the "uint16 command torque" to
% %       apply about the body-frame's y-axis, i.e., the pitch-axis
% % y  -  where "y" stands for yaw, this is the "uint16 command torque" to
% %       apply about the body-frame's z-axis, i.e., the yaw-axis
% %
% % Note: the "/ 2" for the extraction of "r" and "p" above is simply added
% % to minimic the code of the Crazyflie firmware. Presumably the Crazyflie's
% % PID contollers for the body-frame roll and pitch axis are tuned with this
% % factor of "/ 2" appropriately accounted for.
% 
% 
% % Initialise the return variable "cmd_to_apply" to zeros
% % > This can be required so that Simulink knows the expected size
% cmd_to_apply = zeros(4,1);
% 
% % Compute the 16-bit command that should be applied from each motor as per
% % the code from the Crazyflie firmware
% % > For motor 1:
% cmd_to_apply(1,1)  =  cmd1   - r   + p  +  y;
% % > For motor 1:
% cmd_to_apply(2,1)  =  cmd2   - r   - p  -  y;
% % > For motor 1:
% cmd_to_apply(3,1)  =  cmd3   + r   - p  +  y;
% % > For motor 1:
% cmd_to_apply(4,1)  =  cmd4   + r   + p  -  y;

cmd_to_apply = zeros(4,1);

T = cmd1 + cmd2 +cmd3 + cmd4;

tau_x = cmd_for_body_torques_desired(1) / 2;
tau_y = cmd_for_body_torques_desired(2) / 2;
tau_z = cmd_for_body_torques_desired(3);


cmd_to_apply = inv_M*[T;tau_x;tau_y;tau_z];

== matlab function Iris_DeePC_Control_Gazebo_hyper/Quadrotor Model/Measurements/draw sample from multivariate Gaussian for accelerometer ==
  data: std_normal_rand_sample input; rand_sample output; mean_vector input; covariance_matrix_decomposition input
function rand_sample = mvn_accelerometer( std_normal_rand_sample , mean_vector , covariance_matrix_decomposition )


% Compute the multi-variate Gaussian sample from a distirbution with:
% > "mean_vector" as the mean, and
% > "covariance_matrix_decomposition" as the "square root" of the
%    covariance matrix
rand_sample = mean_vector + covariance_matrix_decomposition * std_normal_rand_sample;

== matlab function Iris_DeePC_Control_Gazebo_hyper/Quadrotor Model/Measurements/draw sample from multivariate Gaussian for full state ==
  data: std_normal_rand_sample input; rand_sample output; mean_vector input; covariance_matrix_decomposition input
function rand_sample = mvn_full_state( std_normal_rand_sample , mean_vector , covariance_matrix_decomposition )


% Compute the multi-variate Gaussian sample from a distirbution with:
% > "mean_vector" as the mean, and
% > "covariance_matrix_decomposition" as the "square root" of the
%    covariance matrix
rand_sample = mean_vector + covariance_matrix_decomposition * std_normal_rand_sample;

== matlab function Iris_DeePC_Control_Gazebo_hyper/Quadrotor Model/Measurements/draw sample from multivariate Gaussian for gyroscope ==
  data: std_normal_rand_sample input; rand_sample output; mean_vector input; covariance_matrix_decomposition input
function rand_sample = mvn_gyroscope( std_normal_rand_sample , mean_vector , covariance_matrix_decomposition )


% Compute the multi-variate Gaussian sample from a distirbution with:
% > "mean_vector" as the mean, and
% > "covariance_matrix_decomposition" as the "square root" of the
%    covariance matrix
rand_sample = mean_vector + covariance_matrix_decomposition * std_normal_rand_sample;

== matlab function Iris_DeePC_Control_Gazebo_hyper/Controller/MATLAB Function ==
  data: yawd input; u_virtual input; T output; euler_d output; euler input; mass parameter; accel_g parameter; flag_input_transform_nonlinearity parameter
function [T, euler_d] = input_transform(yawd, u_virtual, euler, mass, accel_g, flag_input_transform_nonlinearity)

T = 0;
euler_d = zeros(3,1);

% Compute pitch, roll and T
Rz = eul2rotm([euler(3,1),0,0],'ZYX');

T_aux = mass * Rz'*(accel_g*[0;0;1] - u_virtual);

if flag_input_transform_nonlinearity
    pitchd = atan2(T_aux(1),T_aux(3));
    rolld = atan2(-T_aux(2),norm(T_aux([1,3])));

%     T = norm(T_aux);
else
    pitchd = T_aux(1);
    rolld = -T_aux(2);

%     T = -u_virtual(3) + mass*accel_g;
end

T = -u_virtual(3) + mass*accel_g;
euler_d = [rolld;pitchd;yawd];

== matlab function Iris_DeePC_Control_Gazebo_hyper/Controller/MATLAB Function1 ==
  data: state_error input; u_virtual output; pp input; xi output; Kp_xy parameter; Kv_xy parameter; Kv_z parameter; Ki_z parameter; Kp_z parameter; Ki_xy parameter
function [u_virtual,xi] = Controller(state_error, pp, Kp_xy, Kv_xy, Kv_z, Ki_z, Kp_z,Ki_xy)

p_err = state_error(1:3);
v_err = state_error(4:6);

u_virtual = zeros(3,1);
xi = zeros(3,1);

% Kv = -4;
% Kp = -4;
% Ki = 0;
% u = Kp*(p_err) + Kv*(v_err) + Ki*pp;
% u_virtual = u(:);

% Kp_xy = - 0.6552/3.6732;
% Kv_xy = - 0.7005/3.6732;
% 
% Kp_z = -0.3120;
% Kv_z = -0.9245;
% Ki = 0;

u_xy = Kv_xy*(v_err(1:2)) + Kp_xy*(p_err(1:2)) + Ki_xy*pp(1:2);

u_z = Kp_z*(p_err(3)) + Kv_z*(v_err(3)) + Ki_z*pp(3);

u_virtual = [u_xy;u_z];

xi = p_err;
